simulink model "task_5_sim"  (R2022b)
settings: Solver=VariableStepAuto  StartTime=0.0  StopTime=20.0  RelTol=1e-3
undefined symbols (not defined in the file or in its folder): A, B, C, KTld5_1, L5_1, r
settings Model: Creator=小灰  LastModifiedBy=小灰

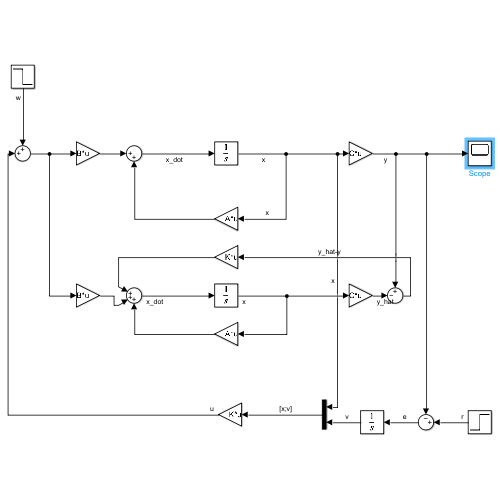
[thumbnail: Simulink's stored preview of the top-level diagram]
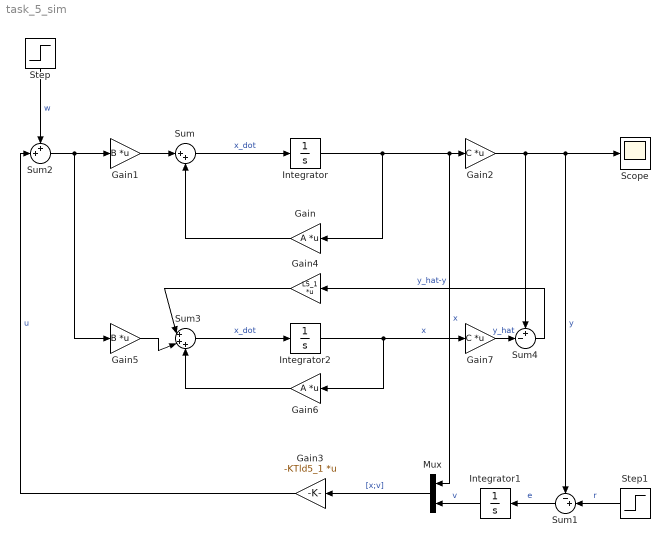
== system task_5_sim ==
  Gain : Gain  Gain=A  Multiplication=Matrix(K*u)
  Gain1 : Gain  Gain=B  Multiplication=Matrix(K*u)
  Gain2 : Gain  Gain=C  Multiplication=Matrix(K*u)
  Gain3 : Gain  Gain=-KTld5_1  Multiplication=Matrix(K*u)
  Gain4 : Gain  Gain=L5_1  Multiplication=Matrix(K*u)
  Gain5 : Gain  Gain=B  Multiplication=Matrix(K*u)
  Gain6 : Gain  Gain=A  Multiplication=Matrix(K*u)
  Gain7 : Gain  Gain=C  Multiplication=Matrix(K*u)
  Integrator : Integrator
  Integrator1 : Integrator
  Integrator2 : Integrator
  Mux : Mux  Inputs=2
  Scope : Scope
  Step : Step  Time=10  Before=[0;0]  After=[-1;1]  SampleTime=0
  Step1 : Step  After=r  SampleTime=0
  Sum : Sum  Inputs=|++
  Sum1 : Sum  Inputs=-+|
  Sum2 : Sum  Inputs=++|
  Sum3 : Sum  Inputs=|+++
  Sum4 : Sum  Inputs=+-|
  wires:
  Sum/1 -> Integrator/1  "x_dot"
  Integrator/1 -> Gain/1, Mux/1, Gain2/1  "x"
  Gain2/1 -> Sum1/1, Scope/1, Sum4/1  "y"
  Mux/1 -> Gain3/1  "[x;v]"
  Sum1/1 -> Integrator1/1  "e"
  Integrator1/1 -> Mux/2  "v"
  Step/1 -> Sum2/1  "w"
  Gain3/1 -> Sum2/2  "u"
  Gain1/1 -> Sum/1
  Sum2/1 -> Gain5/1, Gain1/1
  Gain/1 -> Sum/2
  Step1/1 -> Sum1/2  "r"
  Sum3/1 -> Integrator2/1  "x_dot"
  Integrator2/1 -> Gain6/1, Gain7/1  "x"
  Gain7/1 -> Sum4/2  "y_hat"
  Sum4/1 -> Gain4/1  "y_hat-y"
  Gain6/1 -> Sum3/3
  Gain5/1 -> Sum3/2
  Gain4/1 -> Sum3/1
